simulink model "HC_SRO4"  (R2024b)
settings: Solver=FixedStepAuto  StartTime=0.0  StopTime=inf  RelTol=1e-3  EnableMultiTasking=on
libraries: arduinolib x5, simulink x2, arduinoavrlib x2
settings Model: ExtModeTrigDuration=2  Creator=Tim  LastModifiedBy=Tim
settings SolverCC: AutoInsertRateTranBlk=on
settings OptimizationCC: DefaultParameterBehavior=Inlined  EnhancedBackFolding=on  PassReuseOutputArgsAs=Individual arguments  ZeroExternalMemoryAtStartup=off  ZeroInternalMemoryAtStartup=off  MaxStackSize=64  OptimizeBlockOrder=speed  DifferentSizesBufferReuse=on  OptimizationCustomize=off  EfficientTunableParamExpr=on
settings DebuggingCC: MultiTaskDSMMsg=none  ParameterTunabilityLossMsg=error
settings HardwareCC: ProdBitPerInt=16  ProdBitPerPointer=16  ProdBitPerSizeT=16  ProdBitPerPtrDiffT=16  ProdLargestAtomicFloat=None  ProdWordSize=8  ProdLongLongMode=on  ProdHWDeviceType=Atmel->AVR
settings SFSimCC: MATLABDynamicMemAlloc=off
settings RTWCC: Description=Embedded Coder  SystemTargetFile=ert.tlc  HardwareBoard=Arduino Uno  TemplateMakefile=ert_default_tmf  Toolchain=Arduino AVR  BuildConfiguration=Faster Runs
settings CodeAppCC: ForceParamTrailComments=on  IgnoreCustomStorageClasses=off  OperatorAnnotations=on  SimulinkDataObjDesc=on  SFDataObjDesc=on  InsertBlockDesc=on
settings ERTTargetCC: SupportContinuousTime=on  SupportVariableSizeSignals=on  ExtModeTransport=3  ExtModeStaticAlloc=on  ExtModeAutomaticAllocSize=off  ExtModeStaticAllocSize=250  ExtModeMexFile=ext_xcp  ExtModeIntrfLevel=Level2 - Open

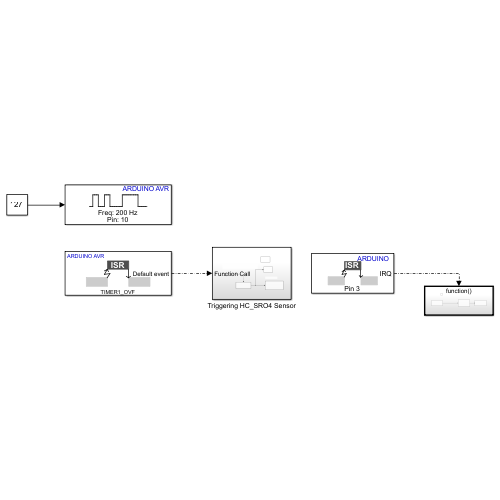
[thumbnail: Simulink's stored preview of the top-level diagram]
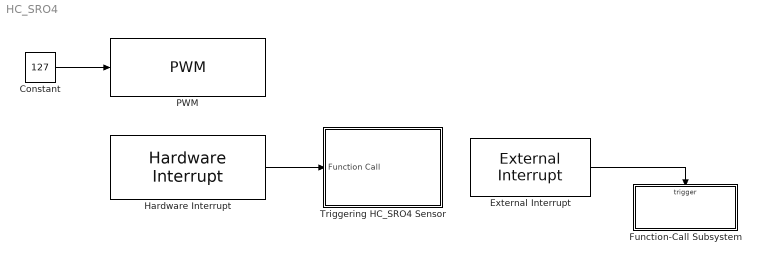
== system HC_SRO4 ==
  Constant : Constant  Value=127
  External Interrupt : arduinolib/External Interrupt  Pin=3  PullUp=off  Mode=CHANGE  InterruptSimulationInput=off
  Function-Call Subsystem : Subsystem  TreatAsAtomicUnit=on
  Hardware Interrupt : arduinoavrlib/Hardware Interrupt  ISRGroup=Timer 1  ISRName=TIMER1_OVF  ISRNumber=7  EventsList={'on','Default event','1'}  SelectedEvents={'Default event'}  TaskPriority=8  DisablePreemption=on  ClearInterruptFlagsAtEndOfEvent=off  HardwareBoard=ARDUINO AVR
  PWM : arduinoavrlib/PWM  pinNumber=10  desiredFrequency=200  achievableFrequency=200  EnableCompareMatchInterrupt=off  EnableOverflowInterrupt=on
  Triggering HC_SRO4 Sensor : Subsystem
  wires:
  Constant/1 -> PWM/1
  Hardware Interrupt/1 -> Triggering HC_SRO4 Sensor/1(Function Call)
  External Interrupt/1 -> Function-Call Subsystem/Trigger

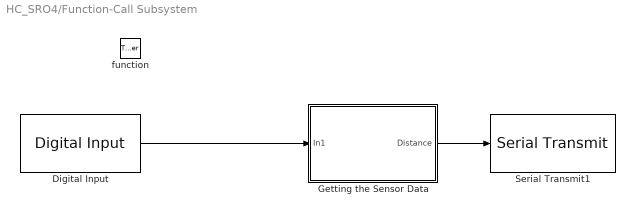
== system HC_SRO4/Function-Call Subsystem ==
  function : TriggerPort  TriggerType=function-call  VariantControl=(inherit)
  Digital Input : arduinolib/Digital Input  pinNumber=4  mode=Default  Direction=input  SampleTime=-1  blockPlatform=arduino
  Getting the Sensor Data : Subsystem
  Serial Transmit1 : arduinolib/Serial Transmit  portNumber=0  sendmode=println  sendformat=Decimal  floatprecision=2  header=[]  terminator=[]  blockPlatform=ARDUINO
  wires:
  Digital Input/1 -> Getting the Sensor Data/1(In1)
  Getting the Sensor Data/1(Distance) -> Serial Transmit1/1

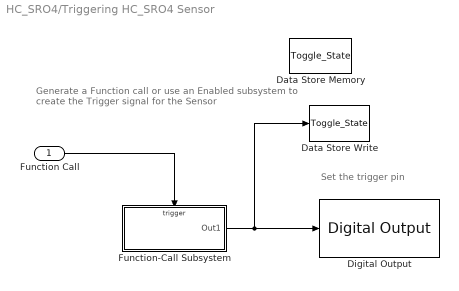
== system HC_SRO4/Triggering HC_SRO4 Sensor ==
  note: Generate a Function call or use an Enabled subsystem to create the Trigger signal for the Sensor
  note: Set the trigger pin
  Function Call : Inport
  Data Store Memory : DataStoreMemory  DataStoreName=Toggle_State  WriteAfterWriteMsg=warning  ShowAdditionalParam=off
  Data Store Write : DataStoreWrite  DataStoreName=Toggle_State  IndexOptions=Index vector (dialog)  Indices=1  OutputSizes=1
  Digital Output : arduinolib/Digital Output  pinNumber=5  Direction=output  blockPlatform=arduino
  Function-Call Subsystem : Subsystem  TreatAsAtomicUnit=on
  wires:
  Function Call/1 -> Function-Call Subsystem/Trigger
  Function-Call Subsystem/1(Out1) -> Data Store Write/1, Digital Output/1

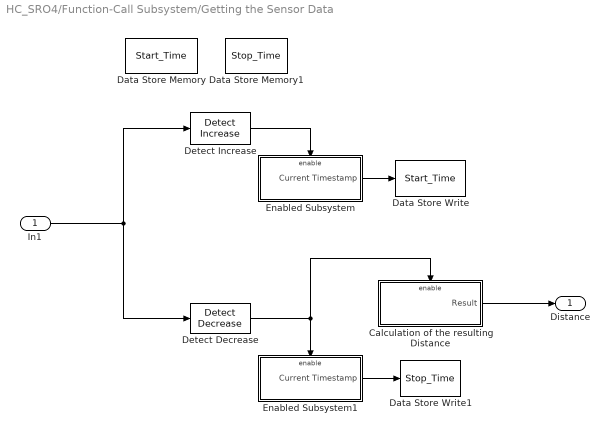
== system HC_SRO4/Function-Call Subsystem/Getting the Sensor Data ==
  In1 : Inport
  Calculation of the resulting Distance : Subsystem  TreatAsAtomicUnit=on
  Data Store Memory : DataStoreMemory  DataStoreName=Start_Time  WriteAfterWriteMsg=warning  ShowAdditionalParam=off
  Data Store Memory1 : DataStoreMemory  DataStoreName=Stop_Time  WriteAfterWriteMsg=warning  ShowAdditionalParam=off
  Data Store Write : DataStoreWrite  DataStoreName=Start_Time  IndexOptions=Index vector (dialog)  Indices=1  OutputSizes=1
  Data Store Write1 : DataStoreWrite  DataStoreName=Stop_Time  IndexOptions=Index vector (dialog)  Indices=1  OutputSizes=1
  Detect Decrease : simulink/Logic and Bit Operations/Detect Decrease  vinit=0.0  OutDataTypeStr=boolean
  Detect Increase : simulink/Logic and Bit Operations/Detect Increase  vinit=0.0  OutDataTypeStr=boolean
  Enabled Subsystem : Subsystem  TreatAsAtomicUnit=on
  Enabled Subsystem1 : Subsystem  TreatAsAtomicUnit=on
  Distance : Outport
  wires:
  In1/1 -> Detect Decrease/1, Detect Increase/1
  Detect Decrease/1 -> Calculation of the resulting Distance/Enable, Enabled Subsystem1/Enable
  Detect Increase/1 -> Enabled Subsystem/Enable
  Enabled Subsystem1/1(Current Timestamp) -> Data Store Write1/1
  Enabled Subsystem/1(Current Timestamp) -> Data Store Write/1
  Calculation of the resulting Distance/1(Result) -> Distance/1

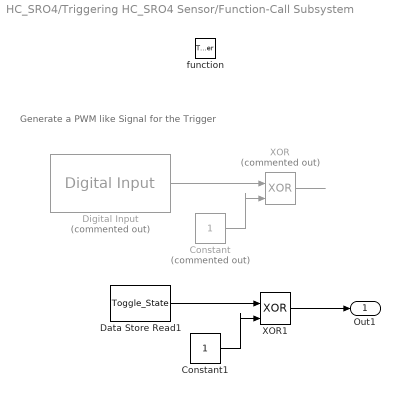
== system HC_SRO4/Triggering HC_SRO4 Sensor/Function-Call Subsystem ==
  note: Generate a PWM like Signal for the Trigger
  function : TriggerPort  TriggerType=function-call  VariantControl=(inherit)
  Constant : Constant  Commented=on
  Constant1 : Constant
  Data Store Read1 : DataStoreRead  DataStoreName=Toggle_State  IndexOptions=Index vector (dialog)  Indices=1  OutputSizes=1
  Digital Input : arduinolib/Digital Input  Commented=on  pinNumber=3  mode=Default  Direction=input  SampleTime=-1  blockPlatform=arduino
  XOR : Logic  Commented=on  Operator=XOR  IconShape=distinctive  AllPortsSameDT=off  OutDataTypeStr=boolean
  XOR1 : Logic  Operator=XOR  IconShape=distinctive  AllPortsSameDT=off  OutDataTypeStr=boolean
  Out1 : Outport
  wires:
  Digital Input/1 -> XOR/1
  Constant/1 -> XOR/2
  XOR/1 -> ?
  Constant1/1 -> XOR1/2
  XOR1/1 -> Out1/1
  Data Store Read1/1 -> XOR1/1

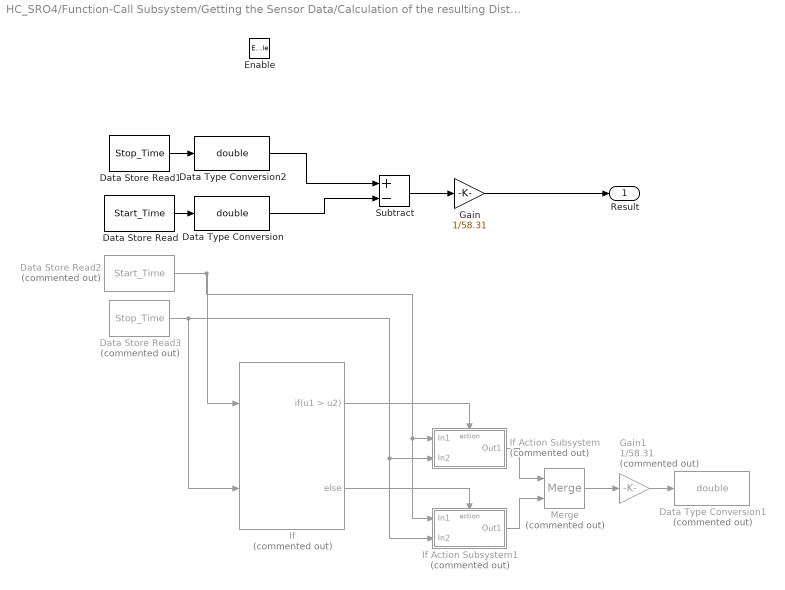
== system HC_SRO4/Function-Call Subsystem/Getting the Sensor Data/Calculation of the resulting Distance ==
  Enable : EnablePort
  Data Store Read : DataStoreRead  DataStoreName=Start_Time  IndexOptions=Index vector (dialog)  Indices=1  OutputSizes=1
  Data Store Read1 : DataStoreRead  DataStoreName=Stop_Time  IndexOptions=Index vector (dialog)  Indices=1  OutputSizes=1
  Data Store Read2 : DataStoreRead  Commented=on  DataStoreName=Start_Time  IndexOptions=Index vector (dialog)  Indices=1  OutputSizes=1
  Data Store Read3 : DataStoreRead  Commented=on  DataStoreName=Stop_Time  IndexOptions=Index vector (dialog)  Indices=1  OutputSizes=1
  Data Type Conversion : DataTypeConversion  OutDataTypeStr=double  SaturateOnIntegerOverflow=off  RndMeth=Floor
  Data Type Conversion1 : DataTypeConversion  Commented=on  OutDataTypeStr=double  SaturateOnIntegerOverflow=off  RndMeth=Floor
  Data Type Conversion2 : DataTypeConversion  OutDataTypeStr=double  SaturateOnIntegerOverflow=off  RndMeth=Floor
  Gain : Gain  Gain=1/58.31
  Gain1 : Gain  Commented=on  Gain=1/58.31
  If : If  Commented=on  NumInputs=2  IfExpression=u1 > u2
  If Action Subsystem : Subsystem  Commented=on  TreatAsAtomicUnit=on
  If Action Subsystem1 : Subsystem  Commented=on  TreatAsAtomicUnit=on
  Merge : Merge  Commented=on
  Subtract : Sum  Inputs=+-
  Result : Outport
  wires:
  Data Store Read1/1 -> Data Type Conversion2/1
  Data Store Read/1 -> Data Type Conversion/1
  Subtract/1 -> Gain/1
  Gain/1 -> Result/1
  Data Store Read2/1 -> If Action Subsystem1/1(In1), If Action Subsystem/1(In1), If/1
  Data Store Read3/1 -> If/2, If Action Subsystem1/2(In2), If Action Subsystem/2(In2)
  If/2 -> If Action Subsystem1/Action
  If/1 -> If Action Subsystem/Action
  If Action Subsystem/1(Out1) -> Merge/1
  If Action Subsystem1/1(Out1) -> Merge/2
  Gain1/1 -> Data Type Conversion1/1
  Merge/1 -> Gain1/1
  Data Type Conversion/1 -> Subtract/2
  Data Type Conversion2/1 -> Subtract/1

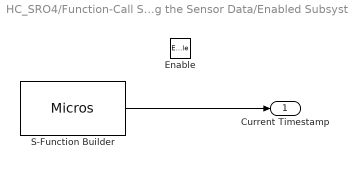
== system HC_SRO4/Function-Call Subsystem/Getting the Sensor Data/Enabled Subsystem ==
  Enable : EnablePort
  S-Function Builder : S-Function  FunctionName=Micros  SFunctionModules=Micros_wrapper.c  SFunctionDeploymentMode=off  EnableBusSupport=off  mask(S-Function Builder){}
      mask help: Simulink:masks:SFunctionBuilder_MD
      mask init:
      | val = [[.9  0.75 0.75 1 1 .9 .9 1]',[1 1 0.75 0.75 .9 .9 1 .9]'];try , sys = get_param(gcb,'SfunBuilderFcnName');if isempty(sys), sys = get_param(gcb,'FunctionName'); end,catch, sys = get_param(gcb,'FunctionName'); end
      settings: CopyFcn=set_param(gcbh,'LinkStatus','none')  OpenFcn=sfunctionwizard(gcbh)
      mask Display:
      | plot(val(:,1),val(:,2))
      | disp(sys)
      | port_label('output',1,sprintf('%s', 'Micros'),'interpreter','tex')
  Current Timestamp : Outport
  wires:
  S-Function Builder/1 -> Current Timestamp/1

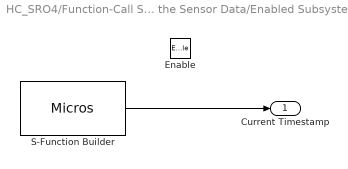
== system HC_SRO4/Function-Call Subsystem/Getting the Sensor Data/Enabled Subsystem1 ==
  Enable : EnablePort
  S-Function Builder : S-Function  FunctionName=Micros  SFunctionModules=Micros_wrapper.c  SFunctionDeploymentMode=off  EnableBusSupport=off  mask(S-Function Builder){}
      mask help: Simulink:masks:SFunctionBuilder_MD
      mask init: same as HC_SRO4/Function-Call Subsystem/Getting the Sensor Data/Enabled Subsystem/S-Function Builder
      settings: CopyFcn=set_param(gcbh,'LinkStatus','none')  OpenFcn=sfunctionwizard(gcbh)
      mask Display:
      | plot(val(:,1),val(:,2))
      | disp(sys)
      | port_label('output',1,sprintf('%s', 'Micros'),'interpreter','tex')
  Current Timestamp : Outport
  wires:
  S-Function Builder/1 -> Current Timestamp/1

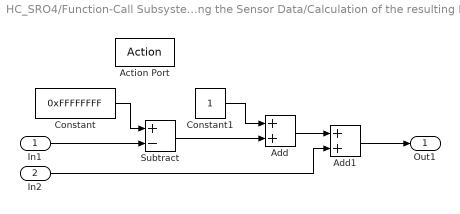
== system HC_SRO4/Function-Call Subsystem/Getting the Sensor Data/Calculation of the resulting Distance/If Action Subsystem ==
  In1 : Inport
  In2 : Inport  Port=2
  Action Port : ActionPort
  Add : Sum
  Add1 : Sum
  Constant : Constant  Value=0xFFFFFFFF
  Constant1 : Constant
  Subtract : Sum  Inputs=+-
  Out1 : Outport
  wires:
  In1/1 -> Subtract/2
  Constant/1 -> Subtract/1
  Subtract/1 -> Add/2
  Constant1/1 -> Add/1
  Add/1 -> Add1/1
  In2/1 -> Add1/2
  Add1/1 -> Out1/1

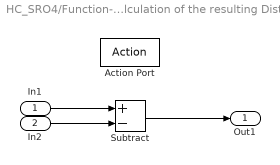
== system HC_SRO4/Function-Call Subsystem/Getting the Sensor Data/Calculation of the resulting Distance/If Action Subsystem1 ==
  In1 : Inport
  In2 : Inport  Port=2
  Action Port : ActionPort
  Subtract : Sum  Inputs=+-
  Out1 : Outport
  wires:
  In1/1 -> Subtract/1
  In2/1 -> Subtract/2
  Subtract/1 -> Out1/1
